simulink model "SystemSISOC"  (Simulink 10.0)
settings: Solver=ode45  StartTime=0.0  StopTime=tend  MaxStep=0.01  RelTol=1e-3  EnableMultiTasking=on
values from neighbouring files (symbols this model uses):
  f = 0.025    [zad1.m]    (also in zad2.m; zad3.m; zad4.m; zad5.m)
  sigma2e = 0.1    [zad6.m]
  TF = 8*Tp    (= 0.4)    [zad6.m]
  Tp = 0.1    [zad1.m]    (also in zad2.m; zad3.m; zad4.m; zad5.m)
libraries: simulink x1
settings Model: Creator=szymo  LastModifiedBy=szymo
settings DataIOCC: LimitDataPoints=on  SignalLoggingSaveFormat=ModelDataLogs
settings OptimizationCC: InitFltsAndDblsToZero=on
settings DebuggingCC: SaveWithParameterizedLinksMsg=none  SignalResolutionControl=TryResolveAllWithWarning  SolverPrmCheckMsg=warning  MultiTaskDSMMsg=warning  MultiTaskCondExecSysMsg=none  FcnCallInpInsideContextMsg=warning
settings SFSimCC: SimUseLocalCustomCode=on  CustomCodeUndefinedFunction=FilterOut
settings RTWCC: RTWUseLocalCustomCode=on
settings GRTTargetCC: TargetFcnLib=ansi_tfl_tmw.mat

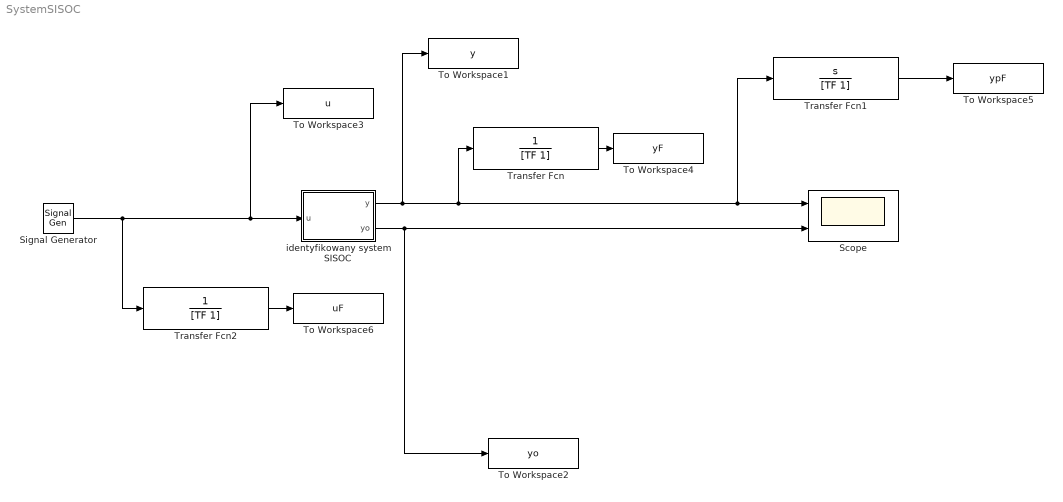
== system SystemSISOC ==
  Scope : Scope  NumInputPorts=2
  Signal Generator : SignalGenerator  WaveForm=square  Frequency=f
  To Workspace1 : ToWorkspace  VariableName=y  SaveFormat=Timeseries  SampleTime=-1
  To Workspace2 : ToWorkspace  VariableName=yo  SaveFormat=Timeseries  SampleTime=-1
  To Workspace3 : ToWorkspace  VariableName=u  SaveFormat=Timeseries  SampleTime=-1
  To Workspace4 : ToWorkspace  VariableName=yF  SaveFormat=Timeseries  SampleTime=-1
  To Workspace5 : ToWorkspace  VariableName=ypF  SaveFormat=Timeseries  SampleTime=-1
  To Workspace6 : ToWorkspace  VariableName=uF  SaveFormat=Timeseries  SampleTime=-1
  Transfer Fcn : TransferFcn  Denominator=[TF 1]
  Transfer Fcn1 : TransferFcn  Numerator=[1 0]  Denominator=[TF 1]
  Transfer Fcn2 : TransferFcn  Denominator=[TF 1]
  identyfikowany system SISOC : Subsystem
  wires:
  Signal Generator/1 -> Transfer Fcn2/1, To Workspace3/1, identyfikowany system SISOC/1(u)
  identyfikowany system SISOC/1(y) -> To Workspace1/1, Transfer Fcn/1, Transfer Fcn1/1, Scope/1
  identyfikowany system SISOC/2(yo) -> To Workspace2/1, Scope/2
  Transfer Fcn/1 -> To Workspace4/1
  Transfer Fcn1/1 -> To Workspace5/1
  Transfer Fcn2/1 -> To Workspace6/1

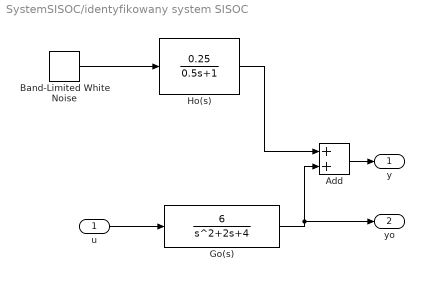
== system SystemSISOC/identyfikowany system SISOC ==
  u : Inport
  Add : Sum
  Band-Limited White Noise : simulink/Sources/Band-Limited White Noise  Cov=[sigma2e]  Ts=Tp*0.1  seed=[2941]
  Go(s) : TransferFcn  Numerator=[6]  Denominator=[1 2 4]
  Ho(s) : TransferFcn  Numerator=[0.25]  Denominator=[0.5 1]
  y : Outport
  yo : Outport  Port=2
  wires:
  Band-Limited White Noise/1 -> Ho(s)/1
  Ho(s)/1 -> Add/1
  Go(s)/1 -> Add/2, yo/1
  Add/1 -> y/1
  u/1 -> Go(s)/1
